simulink model "musyndm3"  (Simulink 3.00)
settings: Solver=ode15s  SolverMode=SingleTasking  StartTime=0.0  StopTime=200  RelTol=1e-3  AbsTol=1e-6
PreLoadFcn:
  | mudata3
undefined symbols (not defined in the file or in its folder): ap, bp, cp, den_i1, den_i2, dp, num_i1, num_i2
settings Model: ExternalInput=[]  SaveTime=off  SaveOutput=off  InitialState=[]  RTWTemplateMakefile=grt_vc.tmf  ExtModeMexFile=ext_comm.c  Creator=greg  LastModifiedBy=David High

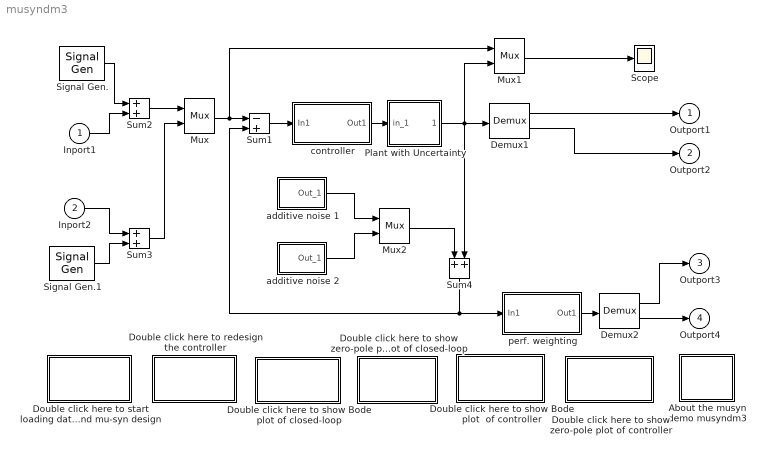
== system musyndm3 ==
  Inport1 : Inport  Port=1  PortWidth=-1  SampleTime=-1  DataType=auto
      settings: SignalType=auto
  Inport2 : Inport  Port=2  PortWidth=-1  SampleTime=-1  DataType=auto
      settings: SignalType=auto
  About the musyn demo musyndm3 : Subsystem
      settings: OpenFcn=clc; more(23); help mudata3; more off; fprintf('\n>>\n');
      mask Display: disp('?')
  Demux1 : Demux  Outputs=2
  Demux2 : Demux  Outputs=2
  Double click here to redesign the controller : Subsystem
      settings: OpenFcn=eval('if ~exist(''mu''),fprintf(''\nMust be licensed for Mu Toolbox\n''), else, fprintf(''\nCtrl_C to abort MuSyn Calculation\n\n''); mudes3; end')
      mask Display: disp('Re-Design')
  Double click here to show Bode plot of closed-loop : Subsystem
      settings: OpenFcn=if ~exist('mu'),fprintf('\nMust be licensed for MuSyn Toolbox\n'),elseif ~exist('g1'),fprintf('\nMust Load Data & Design First\n'),else eval('vplot(''bode'',frsp(g1,logspace(0,4,32)));'); end
      mask Display: disp('Closed-Loop\nBode Plot')
  Double click here to show Bode plot  of controller : Subsystem
      settings: OpenFcn=if ~exist('mu'),fprintf('\nMust be licensed for MuSyn Toolbox\n'),elseif ~exist('k1'), printf('Must Load Data & Design First\n'),else eval('vplot(''bode'',frsp(k1,logspace(0,4,32)));'); end
      mask Display: disp('Controller\nBode Plot')
  Double click here to show zero-pole plot of closed-loop : Subsystem
      settings: OpenFcn=if ~exist('mu'),fprintf('\nMust be licensed for Mu Toolbox\n'),elseif ~exist('g1'), fprintf('Must Load Data & Design First'), else,clf,plot(1:10), eval('[x,y,z,w]=unpck(g1);clf;pzmap(x,y,z,w);clear x y z w');end
      mask Display: disp('Closed-Loop\nZero-Pole\nLocation')
  Double click here to show zero-pole plot of controller : Subsystem
      settings: OpenFcn=if ~exist('mu'),fprintf('\nMust be licensed for Mu Toolbox\n'),elseif ~exist('k1'), fprintf('Must Load Data & Design First'), else,clf,plot(1:10), eval('[x,y,z,w]=unpck(k1);clf;pzmap(x,y,z,w);clear xy z w');end
      mask Display: disp('Controller\nZero-Pole\nLocation')
  Double click here to start loading data and mu-syn design : Subsystem
      settings: OpenFcn=if ~exist('mu'),fprintf('\nMust be licensed for MuSyn Toolbox\n'), else, fprintf('\nLoading Data\nWarning: New data will overlap the original working space data\n>>\n'); mudata3; end
      mask Display: disp('Re-Load\nData')
  Mux : Mux  Inputs=2
      settings: DisplayOption=none
  Mux1 : Mux  Inputs=[2,2]
      settings: DisplayOption=none
  Mux2 : Mux  Inputs=2
      settings: DisplayOption=none
  Plant with Uncertainty : Subsystem
      mask Display: disp('P')
  Scope : Scope
      settings: TickLabels=on  TimeRange=20.000000  YMin=-5  YMax=5  SaveToWorkspace=off  SaveName=ScopeData  DataFormat=Matrix
  Signal Gen. : SignalGenerator  WaveForm=square  Amplitude=1.000000  Frequency=1.000000  Units=rad/sec
  Signal Gen.1 : SignalGenerator  WaveForm=square  Amplitude=3.000000  Frequency=0.500000  Units=rad/sec
  Sum1 : Sum  Inputs=-+  SaturateOnIntegerOverflow=on
  Sum2 : Sum  Inputs=++  SaturateOnIntegerOverflow=on
  Sum3 : Sum  Inputs=++  SaturateOnIntegerOverflow=on
  Sum4 : Sum  Orientation=down  Inputs=++  SaturateOnIntegerOverflow=on
  additive noise 1 : Subsystem  mask{@1=0.001, @2=0.1, @3=79841}
      mask prompts: @1 "Noise Power:"; @2 "Sample Time:"; @3 "Seed"
      mask help:
      | White noise for continuous (s-domain) systems.
      | Band-limited using zero-order-hold.
      mask init:
      | Cov = @1; Ts = @2; seed = @3; r = rand(1,12); r2 = [r(1),r;r,r(12)]; t =[1:13;1:13];
      mask Help: Implemented using white noise into Zero-Order Hold block. The seed and power can be vectors of the same length to produce a vector of white noise sources. For faster simulation, set sample time to the highest value possible but in accordance with the fastest dynamics of system.
      mask Display: plot(t(:),r2(:))
  additive noise 2 : Subsystem  mask{@1=0.001, @2=0.1, @3=123441}
      mask prompts: @1 "Noise Power:"; @2 "Sample Time:"; @3 "Seed"
      mask help:
      | White noise for continuous (s-domain) systems.
      | Band-limited using zero-order-hold.
      mask init:
      | Cov = @1; Ts = @2; seed = @3; r = rand(1,12); r2 = [r(1),r;r,r(12)]; t =[1:13;1:13];
      mask Help: Implemented using white noise into Zero-Order Hold block. The seed and power can be vectors of the same length to produce a vector of white noise sources. For faster simulation, set sample time to the highest value possible but in accordance with the fastest dynamics of system.
      mask Display: plot(t(:),r2(:))
  controller : Subsystem  mask{@1=ak, @2=bk, @3=ck, @4=dk}
      mask prompts: @1 "ak:"; @2 "bk:"; @3 "ck:"; @4 "dk:"
      mask help: H_infty Controller:
      mask init:
      | ak=@1;bk=@2;ck=@3;dk=@4;
      mask Help: . Mask and unmask this block to see how it works.Usinf Mu Analysis and Synthesis Toolbox to design a H_infinity Controller. Change the parameters, see the designed system.
      mask Display: disp('H_infinity\nController')
  perf. weighting : Subsystem  mask{@1=num_o1, @2=den_o1, @3=num_o2, @4=den_o2}
      mask prompts: @1 "numerator of w1:"; @2 "denominator of w1:"; @3 "numerator of w2:"; @4 "denominator of w2:"
      mask help:
      | Performance weighting function:
      | [w1  0]
      | [ 0 w2]
      mask init:
      | [ap,bp,cp,dp]=unpck(daug(nd2sys(@1,@2),nd2sys(@3,@4)));
      mask Help: the weighting function of the plant model.
      mask Display: disp('output\nweighting.')
  "Outport1 " : Outport  Port=1
  "Outport2 " : Outport  Port=2
  Outport3 : Outport  Port=3
  Outport4 : Outport  Port=4
  wires:
  Demux2/2 -> Outport4/1
  Demux2/1 -> Outport3/1
  perf. weighting/1(Out1) -> Demux2/1
  Mux2/1 -> Sum4/1
  additive noise 2/1(Out_1) -> Mux2/2
  Sum4/1 -> Sum1/2, perf. weighting/1(In1)
  Signal Gen.1/1 -> Sum3/2
  Demux1/2 -> "Outport2 "/1
  controller/1(Out1) -> Plant with Uncertainty/1(in_1)
  Signal Gen./1 -> Sum2/1
  Sum2/1 -> Mux/1
  Sum3/1 -> Mux/2
  Inport2/1 -> Sum3/1
  Inport1/1 -> Sum2/2
  Sum1/1 -> controller/1(In1)
  Plant with Uncertainty/1(out_1) -> Demux1/1, Sum4/2, Mux1/2
  additive noise 1/1(Out_1) -> Mux2/1
  Demux1/1 -> "Outport1 "/1
  Mux/1 -> Sum1/1, Mux1/1
  Mux1/1 -> Scope/1

== system musyndm3/About the musyn demo musyndm3 ==

== system musyndm3/Double click here to redesign the controller ==

== system musyndm3/Double click here to show Bode plot of closed-loop ==

== system musyndm3/Double click here to show Bode plot  of controller ==

== system musyndm3/Double click here to show zero-pole plot of closed-loop ==

== system musyndm3/Double click here to show zero-pole plot of controller ==

== system musyndm3/Double click here to start loading data and mu-syn design ==

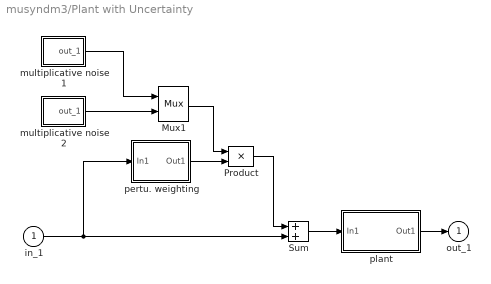
== system musyndm3/Plant with Uncertainty ==
  in_1 : Inport  Port=1  PortWidth=-1  SampleTime=-1  DataType=auto
      settings: SignalType=auto
  Mux1 : Mux  Inputs=2
      settings: DisplayOption=none
  Product : Product  Inputs=2  SaturateOnIntegerOverflow=on
  Sum : Sum  Inputs=++  SaturateOnIntegerOverflow=on
  multiplicative noise 1 : Subsystem  mask{@1=0.02, @2=0.1, @3=68932234}
      mask prompts: @1 "Noise Variance:"; @2 "Sample Time:"; @3 "Seed"
      mask help:
      | White noise for continuous (s-domain) systems.
      | Band-limited using zero-order-hold.
      mask init:
      | Cov = @1; Ts = @2; seed = @3; r = rand(1,12)-0.5; r2 = [r(1),r;r,r(12)]; t =[1:13;1:13];
      mask Help: Implemented using white noise into Zero Order Hold block. For faster simulation set sample time to highest value possible but in accordance with the fastest dynamics of system.
      mask Display: plot(t(:),r2(:))
  multiplicative noise 2 : Subsystem  mask{@1=0.02, @2=0.1, @3=683421}
      mask prompts: @1 "Noise Variance:"; @2 "Sample Time:"; @3 "Seed"
      mask help:
      | White noise for continuous (s-domain) systems.
      | Band-limited using zero-order-hold.
      mask init:
      | Cov = @1; Ts = @2; seed = @3; r = rand(1,12)-0.5; r2 = [r(1),r;r,r(12)]; t =[1:13;1:13];
      mask Help: Implemented using white noise into Zero Order Hold block. For faster simulation set sample time to highest value possible but in accordance with the fastest dynamics of system.
      mask Display: plot(t(:),r2(:))
  pertu. weighting : Subsystem  mask(Transfer Fcn){num_i1=num_i1, den_i1=den_i1, num_i2=num_i2, den_i2=den_i2}
      mask prompts: num_i1 "numerator of w1"; den_i1 "denominator of w1"; num_i2 "numerator of w2"; den_i2 "denominator of w2"
      mask help:
      | Performance weighting function:
      | [ w1  0  ]
      | [ 0   w2 ]
      mask Help: This is the weighting function of the plant model.
      mask Display: disp('   input\nweighting');
  plant : Subsystem  mask{@1=a, @2=b, @3=c, @4=d}
      mask prompts: @1 "a:"; @2 "b:"; @3 "c:"; @4 "d:"
      mask help: state space model:
      mask init:
      | a=@1; b=@2; c=@3; d=@4;
      mask Help: system plant
      mask Display: disp('plant\nmodel')
  out_1 : Outport  Port=1
  wires:
  in_1/1 -> Sum/2, pertu. weighting/1(In1)
  plant/1(Out1) -> out_1/1
  multiplicative noise 2/1(out_1) -> Mux1/2
  Product/1 -> Sum/1
  pertu. weighting/1(Out1) -> Product/2
  Mux1/1 -> Product/1
  Sum/1 -> plant/1(In1)
  multiplicative noise 1/1(out_1) -> Mux1/1

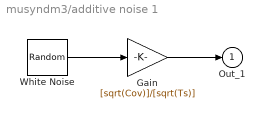
== system musyndm3/additive noise 1 ==
  Gain : Gain  Gain=[sqrt(Cov)]/[sqrt(Ts)]  SaturateOnIntegerOverflow=on
  White Noise : RandomNumber  Mean=0  Variance=1  Seed=seed  SampleTime=Ts
  Out_1 : Outport  Port=1
  wires:
  Gain/1 -> Out_1/1
  White Noise/1 -> Gain/1

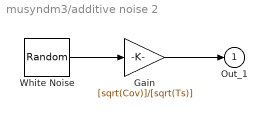
== system musyndm3/additive noise 2 ==
  Gain : Gain  Gain=[sqrt(Cov)]/[sqrt(Ts)]  SaturateOnIntegerOverflow=on
  White Noise : RandomNumber  Mean=0  Variance=1  Seed=seed  SampleTime=Ts
  Out_1 : Outport  Port=1
  wires:
  Gain/1 -> Out_1/1
  White Noise/1 -> Gain/1

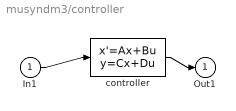
== system musyndm3/controller ==
  In1 : Inport  Port=1  PortWidth=-1  SampleTime=-1  DataType=auto
      settings: SignalType=auto
  controller : StateSpace  A=ak  B=bk  C=ck  D=dk  X0=0
  Out1 : Outport  Port=1
  wires:
  In1/1 -> controller/1
  controller/1 -> Out1/1

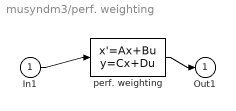
== system musyndm3/perf. weighting ==
  In1 : Inport  Port=1  PortWidth=-1  SampleTime=-1  DataType=auto
      settings: SignalType=auto
  perf. weighting : StateSpace  A=ap  B=bp  C=cp  D=dp  X0=0
  Out1 : Outport  Port=1
  wires:
  In1/1 -> perf. weighting/1
  perf. weighting/1 -> Out1/1

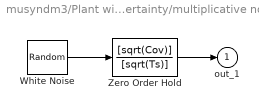
== system musyndm3/Plant with Uncertainty/multiplicative noise 1 ==
  White Noise : RandomNumber  Mean=0  Variance=1  Seed=seed  SampleTime=Ts
  Zero Order Hold : DiscreteTransferFcn  Numerator=[sqrt(Cov)]  Denominator=[sqrt(Ts)]  SampleTime=Ts
  out_1 : Outport  Port=1
  wires:
  Zero Order Hold/1 -> out_1/1
  White Noise/1 -> Zero Order Hold/1

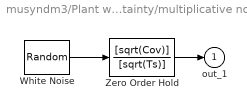
== system musyndm3/Plant with Uncertainty/multiplicative noise 2 ==
  White Noise : RandomNumber  Mean=0  Variance=1  Seed=seed  SampleTime=Ts
  Zero Order Hold : DiscreteTransferFcn  Numerator=[sqrt(Cov)]  Denominator=[sqrt(Ts)]  SampleTime=Ts
  out_1 : Outport  Port=1
  wires:
  Zero Order Hold/1 -> out_1/1
  White Noise/1 -> Zero Order Hold/1

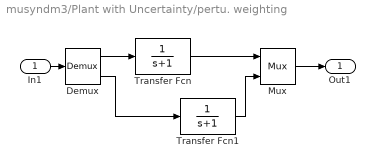
== system musyndm3/Plant with Uncertainty/pertu. weighting ==
  In1 : Inport  Port=1  PortWidth=-1  SampleTime=-1  DataType=auto
      settings: SignalType=auto
  Demux : Demux  Outputs=2
  Mux : Mux  Inputs=2
      settings: DisplayOption=none
  Transfer Fcn : TransferFcn  Numerator=[1]  Denominator=[1 1]
  Transfer Fcn1 : TransferFcn  Numerator=[1]  Denominator=[1 1]
  Out1 : Outport  Port=1
  wires:
  Mux/1 -> Out1/1
  Transfer Fcn1/1 -> Mux/2
  Transfer Fcn/1 -> Mux/1
  In1/1 -> Demux/1
  Demux/2 -> Transfer Fcn1/1
  Demux/1 -> Transfer Fcn/1

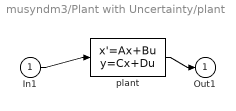
== system musyndm3/Plant with Uncertainty/plant ==
  In1 : Inport  Port=1  PortWidth=-1  SampleTime=-1  DataType=auto
      settings: SignalType=auto
  plant : StateSpace  A=a  B=b  C=c  D=d  X0=0
  Out1 : Outport  Port=1
  wires:
  In1/1 -> plant/1
  plant/1 -> Out1/1
